simulink model "Lab1CEdesen"  (R2019a)
settings: Solver=VariableStepAuto  StartTime=0.0  StopTime=12  RelTol=1e-3
settings Model: Creator=fediu  LastModifiedBy=fediu

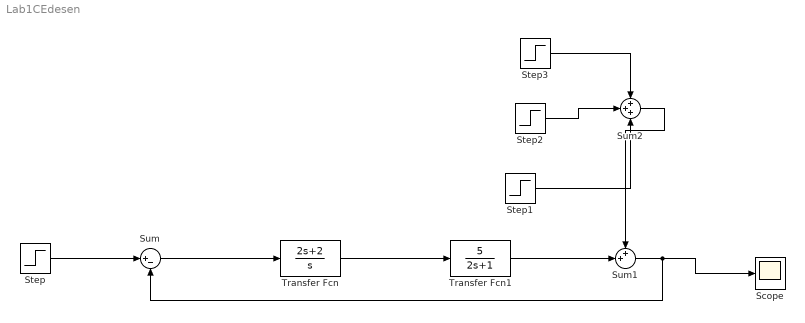
== system Lab1CEdesen ==
  Scope : Scope
  Step : Step  Time=0  SampleTime=0
  Step1 : Step  Time=6  After=0.2  SampleTime=0
  Step2 : Step  Time=8  After=0.1  SampleTime=0
  Step3 : Step  Time=10  After=0.1  SampleTime=0
  Sum : Sum  Inputs=|+-
  Sum1 : Sum  Inputs=++|
  Sum2 : Sum  Inputs=+++
  Transfer Fcn : TransferFcn  Numerator=[2 2]  Denominator=[1 0]
  Transfer Fcn1 : TransferFcn  Numerator=[5]  Denominator=[2 1]
  wires:
  Step/1 -> Sum/1
  Sum1/1 -> Sum/2, Scope/1
  Sum/1 -> Transfer Fcn/1
  Transfer Fcn/1 -> Transfer Fcn1/1
  Transfer Fcn1/1 -> Sum1/2
  Step1/1 -> Sum2/3
  Step2/1 -> Sum2/2
  Step3/1 -> Sum2/1
  Sum2/1 -> Sum1/1
